simulink model "ofdmexample1"  (R2017a)
settings: Solver=FixedStepDiscrete  StartTime=0.0  StopTime=inf  RelTol=1e-3
PostLoadFcn:
  | prm80216d.blkh = []; prm80216d.action = 'init';
  | commwman80216d_init(prm80216d.blkh, prm80216d.action);
  | if isempty(ans), clear ans; end
StartFcn:
  | if isempty(ans), clear ans; end
libraries: commwman80216d_lib x20, dspsigops x16, commcnvcod2 x7, dspsolvers x2, simulink x2, commrflib2 x2, commdigbbndpm3 x1, commblksprivate x1, commofdm x1, commrandsrc3 x1, commsdrhw_v2 x1
Description:
  | IEEE 802.16-2004 WirelessMAN-OFDM PHY Downlink model
settings Model: FPTRunName=Active  ExtModeAutoUpdateStatusClock=off  Creator=The MathWorks, Inc.  LastModifiedBy=max
settings DataIOCC: LimitDataPoints=on  SaveFormat=Array
settings OptimizationCC: ExpressionDepthLimit=2147483647  InitFltsAndDblsToZero=on  EfficientMapNaN2IntZero=off  LifeSpan=inf
settings DebuggingCC: UnderspecifiedInitializationDetection=Classic  MergeDetectMultiDrivingBlocksExec=none  FcnCallInpInsideContextMsg=warning  AllowSymbolicDim=off  StateNameClashWarn=warning  SFUnexpectedBacktrackingDiag=warning  SFNoUnconditionalDefaultTransitionDiag=warning  SFExecutionAtInitializationDiag=none
settings HardwareCC: ProdBitPerPointer=32  ProdBitPerSizeT=32  ProdBitPerPtrDiffT=32  ProdLargestAtomicFloat=None  ProdIntDivRoundTo=Undefined  ProdEndianess=Unspecified  ProdWordSize=32  ProdHWDeviceType=32-bit Generic
settings ModelReferenceCC: PropagateSignalLabelsOutOfModel=off
settings RTWCC: RetainRTWFile=on
settings GRTTargetCC: TargetFcnLib=ansi_tfl_tmw_new.mat  TargetLangStandard=C89/C90 (ANSI)  GeneratePreprocessorConditionals=Disable all  CombineOutputUpdateFcns=off  GRTInterface=on
settings ConfigComp: CovMetricSettings=dw  CovHtmlReporting=on  CovSaveCumulativeToWorkspaceVar=on  CovSaveSingleToWorkspaceVar=on  CovExternalEMLEnable=off  CovSFcnEnable=off

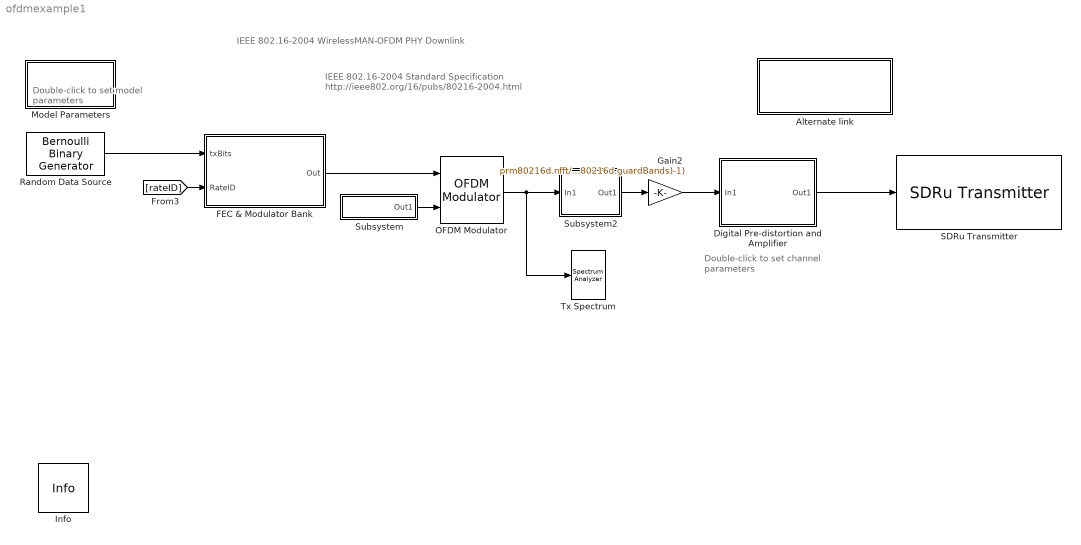
== system ofdmexample1 ==
  note: IEEE 802.16-2004 WirelessMAN-OFDM PHY Downlink
  note: Double-click to set
      | channel parameters
  note: Double-click to
      | set model parameters
  note: IEEE 802.16-2004 Standard Specification
      | http://ieee802.org/16/pubs/80216-2004.html
  Alternate link : Subsystem
      settings: OpenFcn=commwman80216dstbc;
      mask Display: disp('Double-click to open\n link model with\nSpace-Time Block Coding');
  Digital Pre-distortion and Amplifier : Subsystem
      mask Display: disp('Digital\nPre-Distortion and\nNonlinear\nAmplifier')
  FEC & Modulator Bank : Subsystem
      mask Display: disp('FEC & \nModulator Bank');
  Gain2 : Gain  Gain=prm80216d.nfft/sqrt(prm80216d.nfft-sum(prm80216d.guardBands)-1)
  Info : commblksprivate/Info  SystemSampleTime=-1
      settings: SourceProductName=Communications System Toolbox  SourceProductBaseCode=CM
  Model Parameters : Subsystem  mask(Model Parameters){chanBW=3.5, numSym=1, g=1/8, nonlinCtrl=Disabled, dpdCtrl=Disabled, thresh=[4 10 12 19 22 28]}
      mask prompts: chanBW "Channel bandwidth (MHz):"; numSym "Number of OFDM symbols per burst:"; g "Cyclic prefix factor (G):"; nonlinCtrl "Amplifier nonlinearity:"; dpdCtrl "Digital pre-distortion:"; thresh "Low SNR thresholds for rate control (dB):"
      mask help: Specifies model parameters for a simulation run.
      mask init:
      | numPreSym = 1; % number of preamble OFDM symbols
      | 
      | % If the nonlinearity is turned off, then turn off the digital
      | % pre-distortion
      | if nonlinCtrl == 1  % disabled
      |     dpdCtrl = 1;
      | end
      | 
      | myException = commwman80216d_init(gcbh, 'init', chanBW, ...
      |     numSym, numPreSym, g, thresh);
      | 
      | if ~isempty(myException)
      |     errordlg(myException.msg);
      | end
      mask Help: helpview(commdhelp);
      mask TypeOptions g: 1/4 | 1/8 | 1/16 | 1/32
      mask TypeOptions nonlinCtrl: Disabled | Moderate (correctable by pre-distortion) | Severe (uncorrectable by pre-distortion)
      mask Callback nonlinCtrl: commwman80216d_init(gcbh, 'cbShowHidePreDistortion');
      mask TypeOptions dpdCtrl: Disabled | Enabled
      mask Display: disp('Model\nParameters');
  OFDM Modulator : commofdm/OFDM Modulator  FFTLength=prm80216d.nfft  NumGuardBandCarriers=prm80216d.guardBands  InsertDCNull=on  PilotInputPort=on  PilotCarrierIndices=prm80216d.pilotIndices + prm80216d.nfft/2 + 1  CyclicPrefixLength=prm80216d.CPLen  Windowing=off  WindowLength=1  NumSymbols=prm80216d.numOFDMSymbols  NumTransmitAntennas=1  SimulateUsing=Interpreted execution
      settings: SourceProductName=Communications System Toolbox  SourceProductBaseCode=CM
  Random Data Source : commrandsrc3/Bernoulli Binary Generator  ProbabilityOfZero=0.5  SeedSource=Parameter  Seed=61  SampleTime=prm80216d.minBitPeriod  SamplesPerFrame=prm80216d.maxUncBitsPerBlk*prm80216d.numOFDMSymbols  OutputDataType=boolean  SimulateUsing=Interpreted execution
  SDRu Transmitter : commsdrhw_v2/SDRu Transmitter  SourceLibraryInfo="This block requires <a href=\"http://www.mathworks.com/hardware-support/usrp.html\">Communications System Toolbox Support Package for USRP Radio</a>"  rxtx=tx  platform=B210  USRP2_IP='192.168.10.2'  USRP_IP_X300='192.168.10.2'  USRP_IP_X310='192.168.10.2'  USRP_serialNumB200=''  USRP_serialNumB210='30D0D1D'  ChannelMapping=1  centerFrequency=2.484e9  centerFrequencySrc=Dialog  loOffset=0  loOffsetSrc=Dialog  PPSSource=Internal  clockSource=Internal  masterClkRateB200=32e6  masterClkRateB210=8e6  masterClkRateX300=200e6  masterClkRateX310=200e6  masterClkRateParam=8000000  gain=70  gainSrc=Dialog  decimInterp=512  decimInterpSrc=Dialog  TransportDataType=int16  USRP2_IP_NUM=[51 48 68 48 68 49 68]  frameLength=362  outputDatatype=Same as transport data type  overrunUnderrunPort=off  sampleTime=1  dboardInfo=|  HOST_DATA_PORT=30000  HOST_CONTROL_PORT=30001  USRP2_DATA_PORT=32769  USRP2_CONTROL_PORT=32768  bufferMode=Continuous streaming  EnableBurstMode=off  NumFramesInBurst=100  USRP_ID='30D0D1D'
      | dbid: 0
      |           dbName: 'no db found'
      |          freqMin: 0
      |          freqMax: 0
      |          gainMin: 0
      |          gainMax: 0
      |     gainStepSize: 0
      settings: SourceProductName=Communications System Toolbox Support Package for USRP(R) Radio  SourceProductBaseCode=USRP
  Subsystem : Subsystem
      mask Display: disp('Pilot')
  Subsystem2 : Subsystem
      mask Display: disp('Preamble\nPacking');
  Tx Spectrum : SpectrumAnalyzer
  wires:
  Gain2/1 -> Digital Pre-distortion and Amplifier/1(In1)
  Random Data Source/1 -> FEC & Modulator Bank/1(txBits)
  [rateID] -> FEC & Modulator Bank/2(RateID)
  Subsystem/1(Out1) -> OFDM Modulator/2
  OFDM Modulator/1 -> Subsystem2/1(In1), Tx Spectrum/1
  FEC & Modulator Bank/1(Out) -> OFDM Modulator/1
  Subsystem2/1(Out1) -> Gain2/1
  Digital Pre-distortion and Amplifier/1(Out1) -> SDRu Transmitter/1

== system ofdmexample1/Alternate link ==

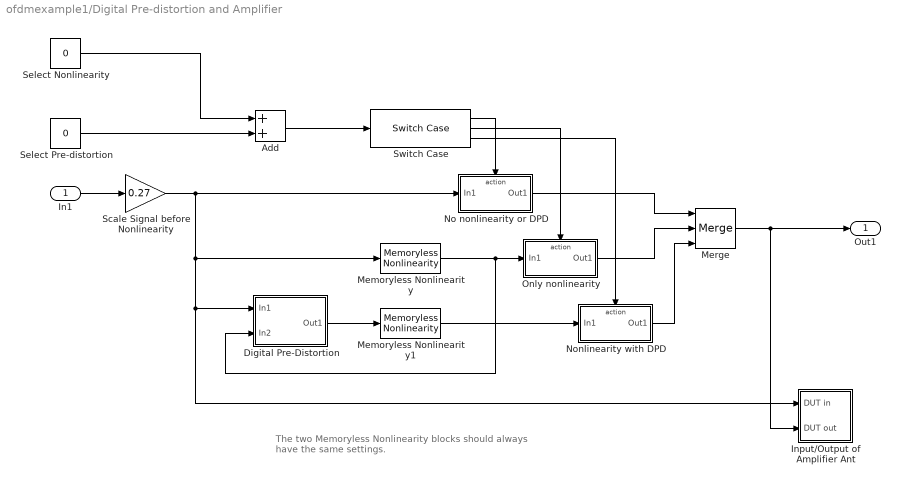
== system ofdmexample1/Digital Pre-distortion and Amplifier ==
  note: The two Memoryless Nonlinearity blocks should always
      | have the same settings.
  In1 : Inport
  Add : Sum
  Digital Pre-Distortion : Subsystem
      mask Display: disp('Digital\nPre-Distortion')
  Input/Output of Amplifier Ant : Subsystem
  Memoryless Nonlinearity : commrflib2/Memoryless Nonlinearity  model_select=Saleh model  linGaindB=0  GindB=0  iip3=30  am2pm=10  LPwrLimAMPM=10  UPwrLimAMPM=inf  amam=[2.1587 1.1517]  ampm=[4.0033 9.1040]  x=[8.1081 1.5413 6.5202 -0.0718]  y=[4.6645 2.0965 10.88 -0.003]  p=0.5  GoutdB=0  vsat=1
      settings: SourceProductName=Communications System Toolbox  SourceProductBaseCode=CM
  Memoryless Nonlinearity1 : commrflib2/Memoryless Nonlinearity  model_select=Saleh model  linGaindB=0  GindB=0  iip3=30  am2pm=10  LPwrLimAMPM=10  UPwrLimAMPM=inf  amam=[2.1587 1.1517]  ampm=[4.0033 9.1040]  x=[8.1081 1.5413 6.5202 -0.0718]  y=[4.6645 2.0965 10.88 -0.003]  p=0.5  GoutdB=0  vsat=1
      settings: SourceProductName=Communications System Toolbox  SourceProductBaseCode=CM
  Merge : Merge  Inputs=3
  No nonlinearity or DPD : Subsystem  TreatAsAtomicUnit=on
  Nonlinearity with DPD : Subsystem  TreatAsAtomicUnit=on
  Only nonlinearity : Subsystem  TreatAsAtomicUnit=on
  Scale Signal before Nonlinearity : Gain  Gain=0.27
  Select Nonlinearity : Constant  Value=0
  Select Pre-distortion : Constant  Value=0
  Switch Case : SwitchCase  CaseConditions={0,1,2}  ShowDefaultCase=off
  Out1 : Outport
  wires:
  Scale Signal before Nonlinearity/1 -> No nonlinearity or DPD/1(In1), Input/Output of Amplifier Ant/1(DUT in), Digital Pre-Distortion/1(In1), Memoryless Nonlinearity/1
  Digital Pre-Distortion/1(Out1) -> Memoryless Nonlinearity1/1
  Select Pre-distortion/1 -> Add/2
  Add/1 -> Switch Case/1
  Select Nonlinearity/1 -> Add/1
  In1/1 -> Scale Signal before Nonlinearity/1
  Memoryless Nonlinearity1/1 -> Nonlinearity with DPD/1(In1)
  Memoryless Nonlinearity/1 -> Only nonlinearity/1(In1), Digital Pre-Distortion/2(In2)
  Merge/1 -> Input/Output of Amplifier Ant/2(DUT out), Out1/1
  Switch Case/1 -> No nonlinearity or DPD/Action
  Switch Case/2 -> Only nonlinearity/Action
  Switch Case/3 -> Nonlinearity with DPD/Action
  No nonlinearity or DPD/1(Out1) -> Merge/1
  Only nonlinearity/1(Out1) -> Merge/2
  Nonlinearity with DPD/1(Out1) -> Merge/3

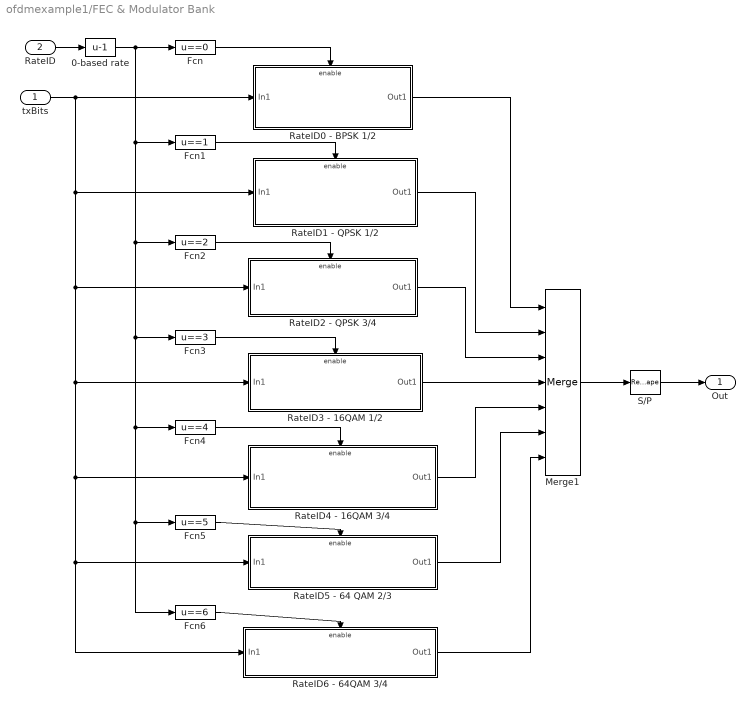
== system ofdmexample1/FEC & Modulator Bank ==
  txBits : Inport
  RateID : Inport  Port=2
  0-based rate : Bias  Bias=-1
  Fcn : Fcn  Expr=u==0
  Fcn1 : Fcn  Expr=u==1
  Fcn2 : Fcn  Expr=u==2
  Fcn3 : Fcn  Expr=u==3
  Fcn4 : Fcn  Expr=u==4
  Fcn5 : Fcn  Expr=u==5
  Fcn6 : Fcn  Expr=u==6
  Merge1 : Merge  Inputs=7
  RateID0 - BPSK 1/2 : Subsystem
  RateID1 - QPSK 1/2 : Subsystem
  RateID2 - QPSK 3/4 : Subsystem
  RateID3 - 16QAM 1/2 : Subsystem
  RateID4 - 16QAM 3/4 : Subsystem
  RateID5 - 64 QAM 2/3 : Subsystem
  RateID6 - 64QAM 3/4 : Subsystem
  S/P : Reshape  OutputDimensionality=Customize  OutputDimensions=[prm80216d.numDataCarriers, prm80216d.numOFDMSymbols]
  Out : Outport
  wires:
  RateID0 - BPSK 1/2/1(Out1) -> Merge1/1
  RateID1 - QPSK 1/2/1(Out1) -> Merge1/2
  RateID2 - QPSK 3/4/1(Out1) -> Merge1/3
  RateID3 - 16QAM 1/2/1(Out1) -> Merge1/4
  RateID4 - 16QAM 3/4/1(Out1) -> Merge1/5
  RateID5 - 64 QAM 2/3/1(Out1) -> Merge1/6
  RateID6 - 64QAM 3/4/1(Out1) -> Merge1/7
  txBits/1 -> RateID5 - 64 QAM 2/3/1(In1), RateID6 - 64QAM 3/4/1(In1), RateID4 - 16QAM 3/4/1(In1), RateID3 - 16QAM 1/2/1(In1), RateID2 - QPSK 3/4/1(In1), RateID1 - QPSK 1/2/1(In1), RateID0 - BPSK 1/2/1(In1)
  RateID/1 -> 0-based rate/1
  Fcn/1 -> RateID0 - BPSK 1/2/Enable
  Fcn1/1 -> RateID1 - QPSK 1/2/Enable
  Fcn2/1 -> RateID2 - QPSK 3/4/Enable
  Fcn3/1 -> RateID3 - 16QAM 1/2/Enable
  Fcn4/1 -> RateID4 - 16QAM 3/4/Enable
  Fcn5/1 -> RateID5 - 64 QAM 2/3/Enable
  Fcn6/1 -> RateID6 - 64QAM 3/4/Enable
  0-based rate/1 -> Fcn4/1, Fcn5/1, Fcn6/1, Fcn3/1, Fcn2/1, Fcn1/1, Fcn/1
  Merge1/1 -> S/P/1
  S/P/1 -> Out/1

== system ofdmexample1/Model Parameters ==
  note: This subsystem is empty.
      | It is used for setting parameter values (in the mask).

== system ofdmexample1/Subsystem ==
  Gain{,1,3..4} (4 alike) : Gain  Gain=-1
  Input Packing : Concatenate  NumInputs=8  Mode=Multidimensional array
  Pilots : commwman80216d_lib/Pilot Generator  link=Downlink  ts=prm80216d.maxUncBitsPerBlk*prm80216d.minBitPeriod  numSym=prm80216d.numOFDMSymbols  shift=prm80216d.numPreamOFDMSymbols
      settings: SourceProductName=Communications System Toolbox  SourceProductBaseCode=CM
  Out1 : Outport
  wires:
  Gain/1 -> Input Packing/4
  Pilots/1 -> Input Packing/1, Gain1/1, Input Packing/3, Gain/1, Gain3/1, Gain4/1, Input Packing/7, Input Packing/8
  Gain3/1 -> Input Packing/5
  Gain1/1 -> Input Packing/2
  Gain4/1 -> Input Packing/6
  Input Packing/1 -> Out1/1

== system ofdmexample1/Subsystem2 ==
  In1 : Inport
  Insert Preamble : Concatenate  Mode=Multidimensional array
  Subsystem1 : Subsystem
      mask Display: disp('Preamble')
  Out1 : Outport
  wires:
  In1/1 -> Insert Preamble/2
  Insert Preamble/1 -> Out1/1
  Subsystem1/1(Out) -> Insert Preamble/1

== system ofdmexample1/Digital Pre-distortion and Amplifier/Digital Pre-Distortion ==
  In1 : Inport
  In2 : Inport  Port=2
  Distortion compensation : Subsystem
  Parameter Estimation : Subsystem
  Out1 : Outport
  wires:
  In1/1 -> Distortion compensation/3(In), Parameter Estimation/1(DUT Input)
  Parameter Estimation/1(c) -> Distortion compensation/1(c)
  Parameter Estimation/2(d) -> Distortion compensation/2(d)
  Distortion compensation/1(Pre-distorted Signal) -> Out1/1
  In2/1 -> Parameter Estimation/2(DUT Output)

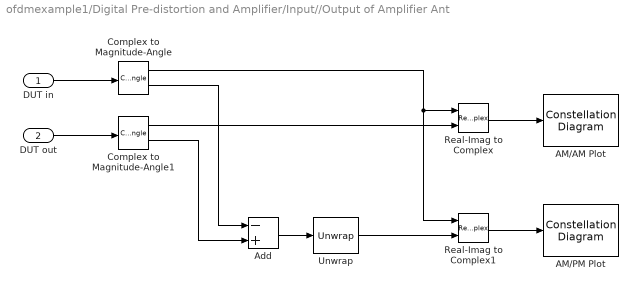
== system ofdmexample1/Digital Pre-distortion and Amplifier/Input//Output of Amplifier Ant ==
  DUT in : Inport
  DUT out : Inport  Port=2
  AM/AM Plot : ConstellationDiagram  Tag=ScatterPlot
  AM/PM Plot : ConstellationDiagram  Tag=ScatterPlot
  Add : Sum  Inputs=-+
  Complex to Magnitude-Angle : ComplexToMagnitudeAngle
  Complex to Magnitude-Angle1 : ComplexToMagnitudeAngle
  Real-Imag to Complex : RealImagToComplex
  Real-Imag to Complex1 : RealImagToComplex
  Unwrap : dspsigops/Unwrap  tol=pi  InputProcessing=Columns as channels (frame based)  running=on
  wires:
  Complex to Magnitude-Angle/1 -> Real-Imag to Complex/1, Real-Imag to Complex1/1
  Complex to Magnitude-Angle1/1 -> Real-Imag to Complex/2
  Real-Imag to Complex/1 -> AM/AM Plot/1
  Real-Imag to Complex1/1 -> AM/PM Plot/1
  DUT in/1 -> Complex to Magnitude-Angle/1
  DUT out/1 -> Complex to Magnitude-Angle1/1
  Complex to Magnitude-Angle1/2 -> Add/2
  Complex to Magnitude-Angle/2 -> Add/1
  Add/1 -> Unwrap/1
  Unwrap/1 -> Real-Imag to Complex1/2

== system ofdmexample1/Digital Pre-distortion and Amplifier/No nonlinearity or DPD ==
  In1 : Inport
  Action Port : ActionPort  ActionType=case
  Out1 : Outport
  wires:
  In1/1 -> Out1/1

== system ofdmexample1/Digital Pre-distortion and Amplifier/Nonlinearity with DPD ==
  In1 : Inport
  Action Port : ActionPort  ActionType=case
  Out1 : Outport
  wires:
  In1/1 -> Out1/1

== system ofdmexample1/Digital Pre-distortion and Amplifier/Only nonlinearity ==
  In1 : Inport
  Action Port : ActionPort  ActionType=case
  Out1 : Outport
  wires:
  In1/1 -> Out1/1

== system ofdmexample1/FEC & Modulator Bank/RateID0 - BPSK 1//2 ==
  In1 : Inport
  Enable : EnablePort  PropagateVarSize=During execution
  BPSK Modulator : commdigbbndpm3/BPSK Modulator Baseband  Ph=0  outDtype=double  outWordLen=16  outUDDataType=sfix(16)  outFracLenMode=Best precision  outFracLen=15  outDataTypeStr=double  outLastDataTypeStr=double
  Convolutional Encoder : commcnvcod2/Convolutional Encoder  trellis=poly2trellis(7, [171 133])  opMode=Truncated (reset every frame)  DelayedResetAction=off  hasIniStPort=off  hasFinStPort=off  usePuncVector=off  punctureVector=[1 0 1]  reset=Unused parameter value
      settings: SourceProductName=Communications System Toolbox  SourceProductBaseCode=CM
  Interleaver : commwman80216d_lib/Interleaver  numSubCh=16  Ncbps1=192  Ncbps2=96  Ncbps3=48  Ncbps4=96  Ncbps5=12  Ncpc=1  numSym=prm80216d.numOFDMSymbols
      settings: SourceProductName=Communications System Toolbox  SourceProductBaseCode=CM
  Select Bits : dspsigops/Pad  padAlong=Columns  dimsToPad=1  valSrc=Specify via dialog  padVal=0  spec=Output size  padNumOutRowsSpecMethod=User-specified  numOutRows=prm80216d.uncBlkSize(1)*8*prm80216d.numOFDMSymbols - 8  padNumOutColsSpecMethod=User-specified  numOutCols=1  isVarDimsMode=off  padBeginning=0  padEnd=0  outSizeMode=User-specified  outSize=1  padSigAt=End  trunc_flag=None  roundingMode=Floor  overflowMode=off  truncOrWrapMode=Truncate  wrap_flag=None
      settings: AttributesFormatString=\n  SourceProductName=DSP System Toolbox  SourceProductBaseCode=DS
  Zero pad tail byte : dspsigops/Pad  padAlong=Columns  dimsToPad=1  valSrc=Specify via dialog  padVal=0  spec=Output size  padNumOutRowsSpecMethod=User-specified  numOutRows=prm80216d.uncBlkSize(1)*8*prm80216d.numOFDMSymbols  padNumOutColsSpecMethod=User-specified  numOutCols=1  isVarDimsMode=off  padBeginning=0  padEnd=0  outSizeMode=User-specified  outSize=1  padSigAt=End  trunc_flag=None  roundingMode=Floor  overflowMode=off  truncOrWrapMode=Truncate  wrap_flag=None
      settings: AttributesFormatString=\n  SourceProductName=DSP System Toolbox  SourceProductBaseCode=DS
  Out1 : Outport
  wires:
  Convolutional Encoder/1 -> Interleaver/1
  Interleaver/1 -> BPSK Modulator/1
  In1/1 -> Select Bits/1
  BPSK Modulator/1 -> Out1/1
  Select Bits/1 -> Zero pad tail byte/1
  Zero pad tail byte/1 -> Convolutional Encoder/1

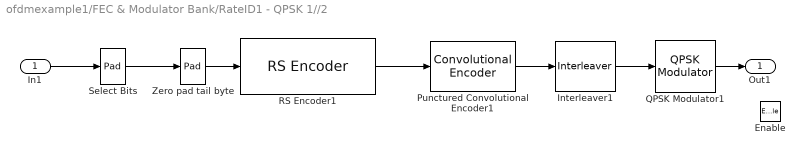
== system ofdmexample1/FEC & Modulator Bank/RateID1 - QPSK 1//2 ==
  In1 : Inport
  Enable : EnablePort  PropagateVarSize=During execution
  Interleaver1 : commwman80216d_lib/Interleaver  numSubCh=16  Ncbps1=384  Ncbps2=96  Ncbps3=48  Ncbps4=96  Ncbps5=12  Ncpc=2  numSym=prm80216d.numOFDMSymbols
      settings: SourceProductName=Communications System Toolbox  SourceProductBaseCode=CM
  Punctured Convolutional Encoder1 : commcnvcod2/Convolutional Encoder  trellis=poly2trellis(7, [171 133])  opMode=Truncated (reset every frame)  DelayedResetAction=off  hasIniStPort=off  hasFinStPort=off  usePuncVector=on  punctureVector=reshape([1 0;1 1],4,1)  reset=Unused parameter value
      settings: SourceProductName=Communications System Toolbox  SourceProductBaseCode=CM
  QPSK Modulator1 : commwman80216d_lib/QPSK Modulator  SystemSampleTime=-1
      settings: SourceProductName=Communications System Toolbox  SourceProductBaseCode=CM
  RS Encoder1 : commwman80216d_lib/RS Encoder  N=32  K=24  numSym=prm80216d.numOFDMSymbols
      settings: SourceProductName=Communications System Toolbox  SourceProductBaseCode=CM
  Select Bits : dspsigops/Pad  padAlong=Columns  dimsToPad=1  valSrc=Specify via dialog  padVal=0  spec=Output size  padNumOutRowsSpecMethod=User-specified  numOutRows=prm80216d.uncBlkSize(2)*8*prm80216d.numOFDMSymbols - 8  padNumOutColsSpecMethod=User-specified  numOutCols=1  isVarDimsMode=off  padBeginning=0  padEnd=0  outSizeMode=User-specified  outSize=1  padSigAt=End  trunc_flag=None  roundingMode=Floor  overflowMode=off  truncOrWrapMode=Truncate  wrap_flag=None
      settings: AttributesFormatString=\n  SourceProductName=DSP System Toolbox  SourceProductBaseCode=DS
  Zero pad tail byte : dspsigops/Pad  padAlong=Columns  dimsToPad=1  valSrc=Specify via dialog  padVal=0  spec=Output size  padNumOutRowsSpecMethod=User-specified  numOutRows=prm80216d.uncBlkSize(2)*8*prm80216d.numOFDMSymbols  padNumOutColsSpecMethod=User-specified  numOutCols=1  isVarDimsMode=off  padBeginning=0  padEnd=0  outSizeMode=User-specified  outSize=1  padSigAt=End  trunc_flag=None  roundingMode=Floor  overflowMode=off  truncOrWrapMode=Truncate  wrap_flag=None
      settings: AttributesFormatString=\n  SourceProductName=DSP System Toolbox  SourceProductBaseCode=DS
  Out1 : Outport
  wires:
  RS Encoder1/1 -> Punctured Convolutional Encoder1/1
  Punctured Convolutional Encoder1/1 -> Interleaver1/1
  Interleaver1/1 -> QPSK Modulator1/1
  In1/1 -> Select Bits/1
  QPSK Modulator1/1 -> Out1/1
  Select Bits/1 -> Zero pad tail byte/1
  Zero pad tail byte/1 -> RS Encoder1/1

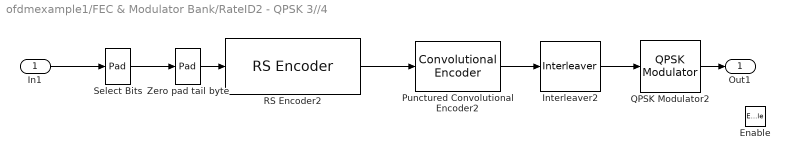
== system ofdmexample1/FEC & Modulator Bank/RateID2 - QPSK 3//4 ==
  In1 : Inport
  Enable : EnablePort  PropagateVarSize=During execution
  Interleaver2 : commwman80216d_lib/Interleaver  numSubCh=16  Ncbps1=384  Ncbps2=96  Ncbps3=48  Ncbps4=96  Ncbps5=12  Ncpc=2  numSym=prm80216d.numOFDMSymbols
      settings: SourceProductName=Communications System Toolbox  SourceProductBaseCode=CM
  Punctured Convolutional Encoder2 : commcnvcod2/Convolutional Encoder  trellis=poly2trellis(7, [171 133])  opMode=Truncated (reset every frame)  DelayedResetAction=off  hasIniStPort=off  hasFinStPort=off  usePuncVector=on  punctureVector=reshape([1 0 1 0 1;1 1 0 1 0],10,1)  reset=Unused parameter value
      settings: SourceProductName=Communications System Toolbox  SourceProductBaseCode=CM
  QPSK Modulator2 : commwman80216d_lib/QPSK Modulator  SystemSampleTime=-1
      settings: SourceProductName=Communications System Toolbox  SourceProductBaseCode=CM
  RS Encoder2 : commwman80216d_lib/RS Encoder  N=40  K=36  numSym=prm80216d.numOFDMSymbols
      settings: SourceProductName=Communications System Toolbox  SourceProductBaseCode=CM
  Select Bits : dspsigops/Pad  padAlong=Columns  dimsToPad=1  valSrc=Specify via dialog  padVal=0  spec=Output size  padNumOutRowsSpecMethod=User-specified  numOutRows=prm80216d.uncBlkSize(3)*8*prm80216d.numOFDMSymbols - 8  padNumOutColsSpecMethod=User-specified  numOutCols=1  isVarDimsMode=off  padBeginning=0  padEnd=0  outSizeMode=User-specified  outSize=1  padSigAt=End  trunc_flag=None  roundingMode=Floor  overflowMode=off  truncOrWrapMode=Truncate  wrap_flag=None
      settings: AttributesFormatString=\n  SourceProductName=DSP System Toolbox  SourceProductBaseCode=DS
  Zero pad tail byte : dspsigops/Pad  padAlong=Columns  dimsToPad=1  valSrc=Specify via dialog  padVal=0  spec=Output size  padNumOutRowsSpecMethod=User-specified  numOutRows=prm80216d.uncBlkSize(3)*8*prm80216d.numOFDMSymbols  padNumOutColsSpecMethod=User-specified  numOutCols=1  isVarDimsMode=off  padBeginning=0  padEnd=0  outSizeMode=User-specified  outSize=1  padSigAt=End  trunc_flag=None  roundingMode=Floor  overflowMode=off  truncOrWrapMode=Truncate  wrap_flag=None
      settings: AttributesFormatString=\n  SourceProductName=DSP System Toolbox  SourceProductBaseCode=DS
  Out1 : Outport
  wires:
  RS Encoder2/1 -> Punctured Convolutional Encoder2/1
  Punctured Convolutional Encoder2/1 -> Interleaver2/1
  Interleaver2/1 -> QPSK Modulator2/1
  In1/1 -> Select Bits/1
  QPSK Modulator2/1 -> Out1/1
  Select Bits/1 -> Zero pad tail byte/1
  Zero pad tail byte/1 -> RS Encoder2/1

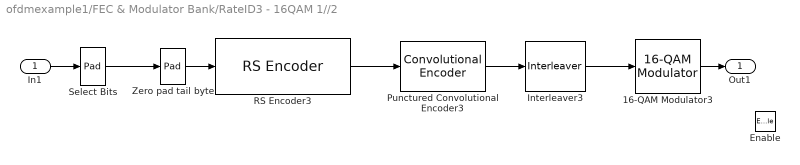
== system ofdmexample1/FEC & Modulator Bank/RateID3 - 16QAM 1//2 ==
  In1 : Inport
  Enable : EnablePort  PropagateVarSize=During execution
  16-QAM Modulator3 : commwman80216d_lib/16-QAM Modulator  SystemSampleTime=-1
      settings: SourceProductName=Communications System Toolbox  SourceProductBaseCode=CM
  Interleaver3 : commwman80216d_lib/Interleaver  numSubCh=16  Ncbps1=768  Ncbps2=96  Ncbps3=48  Ncbps4=96  Ncbps5=12  Ncpc=4  numSym=prm80216d.numOFDMSymbols
      settings: SourceProductName=Communications System Toolbox  SourceProductBaseCode=CM
  Punctured Convolutional Encoder3 : commcnvcod2/Convolutional Encoder  trellis=poly2trellis(7, [171 133])  opMode=Truncated (reset every frame)  DelayedResetAction=off  hasIniStPort=off  hasFinStPort=off  usePuncVector=on  punctureVector=reshape([1 0;1 1],4,1)  reset=Unused parameter value
      settings: SourceProductName=Communications System Toolbox  SourceProductBaseCode=CM
  RS Encoder3 : commwman80216d_lib/RS Encoder  N=64  K=48  numSym=prm80216d.numOFDMSymbols
      settings: SourceProductName=Communications System Toolbox  SourceProductBaseCode=CM
  Select Bits : dspsigops/Pad  padAlong=Columns  dimsToPad=1  valSrc=Specify via dialog  padVal=0  spec=Output size  padNumOutRowsSpecMethod=User-specified  numOutRows=prm80216d.uncBlkSize(4)*8*prm80216d.numOFDMSymbols - 8  padNumOutColsSpecMethod=User-specified  numOutCols=1  isVarDimsMode=off  padBeginning=0  padEnd=0  outSizeMode=User-specified  outSize=1  padSigAt=End  trunc_flag=None  roundingMode=Floor  overflowMode=off  truncOrWrapMode=Truncate  wrap_flag=None
      settings: AttributesFormatString=\n  SourceProductName=DSP System Toolbox  SourceProductBaseCode=DS
  Zero pad tail byte : dspsigops/Pad  padAlong=Columns  dimsToPad=1  valSrc=Specify via dialog  padVal=0  spec=Output size  padNumOutRowsSpecMethod=User-specified  numOutRows=prm80216d.uncBlkSize(4)*8*prm80216d.numOFDMSymbols  padNumOutColsSpecMethod=User-specified  numOutCols=1  isVarDimsMode=off  padBeginning=0  padEnd=0  outSizeMode=User-specified  outSize=1  padSigAt=End  trunc_flag=None  roundingMode=Floor  overflowMode=off  truncOrWrapMode=Truncate  wrap_flag=None
      settings: AttributesFormatString=\n  SourceProductName=DSP System Toolbox  SourceProductBaseCode=DS
  Out1 : Outport
  wires:
  RS Encoder3/1 -> Punctured Convolutional Encoder3/1
  Punctured Convolutional Encoder3/1 -> Interleaver3/1
  Interleaver3/1 -> 16-QAM Modulator3/1
  In1/1 -> Select Bits/1
  16-QAM Modulator3/1 -> Out1/1
  Select Bits/1 -> Zero pad tail byte/1
  Zero pad tail byte/1 -> RS Encoder3/1

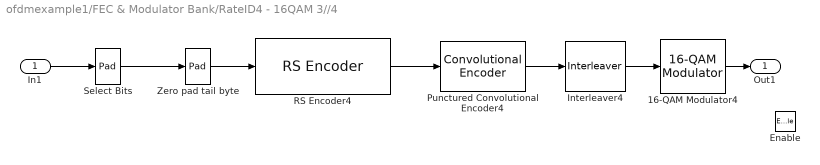
== system ofdmexample1/FEC & Modulator Bank/RateID4 - 16QAM 3//4 ==
  In1 : Inport
  Enable : EnablePort  PropagateVarSize=During execution
  16-QAM Modulator4 : commwman80216d_lib/16-QAM Modulator  SystemSampleTime=-1
      settings: SourceProductName=Communications System Toolbox  SourceProductBaseCode=CM
  Interleaver4 : commwman80216d_lib/Interleaver  numSubCh=16  Ncbps1=768  Ncbps2=96  Ncbps3=48  Ncbps4=96  Ncbps5=12  Ncpc=4  numSym=prm80216d.numOFDMSymbols
      settings: SourceProductName=Communications System Toolbox  SourceProductBaseCode=CM
  Punctured Convolutional Encoder4 : commcnvcod2/Convolutional Encoder  trellis=poly2trellis(7, [171 133])  opMode=Truncated (reset every frame)  DelayedResetAction=off  hasIniStPort=off  hasFinStPort=off  usePuncVector=on  punctureVector=reshape([1 0 1 0 1;1 1 0 1 0],10,1)  reset=Unused parameter value
      settings: SourceProductName=Communications System Toolbox  SourceProductBaseCode=CM
  RS Encoder4 : commwman80216d_lib/RS Encoder  N=80  K=72  numSym=prm80216d.numOFDMSymbols
      settings: SourceProductName=Communications System Toolbox  SourceProductBaseCode=CM
  Select Bits : dspsigops/Pad  padAlong=Columns  dimsToPad=1  valSrc=Specify via dialog  padVal=0  spec=Output size  padNumOutRowsSpecMethod=User-specified  numOutRows=prm80216d.uncBlkSize(5)*8*prm80216d.numOFDMSymbols - 8  padNumOutColsSpecMethod=User-specified  numOutCols=1  isVarDimsMode=off  padBeginning=0  padEnd=0  outSizeMode=User-specified  outSize=1  padSigAt=End  trunc_flag=None  roundingMode=Floor  overflowMode=off  truncOrWrapMode=Truncate  wrap_flag=None
      settings: AttributesFormatString=\n  SourceProductName=DSP System Toolbox  SourceProductBaseCode=DS
  Zero pad tail byte : dspsigops/Pad  padAlong=Columns  dimsToPad=1  valSrc=Specify via dialog  padVal=0  spec=Output size  padNumOutRowsSpecMethod=User-specified  numOutRows=prm80216d.uncBlkSize(5)*8*prm80216d.numOFDMSymbols  padNumOutColsSpecMethod=User-specified  numOutCols=1  isVarDimsMode=off  padBeginning=0  padEnd=0  outSizeMode=User-specified  outSize=1  padSigAt=End  trunc_flag=None  roundingMode=Floor  overflowMode=off  truncOrWrapMode=Truncate  wrap_flag=None
      settings: AttributesFormatString=\n  SourceProductName=DSP System Toolbox  SourceProductBaseCode=DS
  Out1 : Outport
  wires:
  RS Encoder4/1 -> Punctured Convolutional Encoder4/1
  Punctured Convolutional Encoder4/1 -> Interleaver4/1
  Interleaver4/1 -> 16-QAM Modulator4/1
  In1/1 -> Select Bits/1
  16-QAM Modulator4/1 -> Out1/1
  Select Bits/1 -> Zero pad tail byte/1
  Zero pad tail byte/1 -> RS Encoder4/1

== system ofdmexample1/FEC & Modulator Bank/RateID5 - 64 QAM 2//3 ==
  In1 : Inport
  Enable : EnablePort  PropagateVarSize=During execution
  64-QAM Modulator5 : commwman80216d_lib/64-QAM Modulator  SystemSampleTime=-1
      settings: SourceProductName=Communications System Toolbox  SourceProductBaseCode=CM
  Interleaver5 : commwman80216d_lib/Interleaver  numSubCh=16  Ncbps1=1152  Ncbps2=96  Ncbps3=48  Ncbps4=96  Ncbps5=12  Ncpc=6  numSym=prm80216d.numOFDMSymbols
      settings: SourceProductName=Communications System Toolbox  SourceProductBaseCode=CM
  Punctured Convolutional Encoder5 : commcnvcod2/Convolutional Encoder  trellis=poly2trellis(7, [171 133])  opMode=Truncated (reset every frame)  DelayedResetAction=off  hasIniStPort=off  hasFinStPort=off  usePuncVector=on  punctureVector=reshape([1 0 1;1 1 0 ],6,1)  reset=Unused parameter value
      settings: SourceProductName=Communications System Toolbox  SourceProductBaseCode=CM
  RS Encoder5 : commwman80216d_lib/RS Encoder  N=108  K=96  numSym=prm80216d.numOFDMSymbols
      settings: SourceProductName=Communications System Toolbox  SourceProductBaseCode=CM
  Select Bits : dspsigops/Pad  padAlong=Columns  dimsToPad=1  valSrc=Specify via dialog  padVal=0  spec=Output size  padNumOutRowsSpecMethod=User-specified  numOutRows=prm80216d.uncBlkSize(6)*8*prm80216d.numOFDMSymbols - 8  padNumOutColsSpecMethod=User-specified  numOutCols=1  isVarDimsMode=off  padBeginning=0  padEnd=0  outSizeMode=User-specified  outSize=1  padSigAt=End  trunc_flag=None  roundingMode=Floor  overflowMode=off  truncOrWrapMode=Truncate  wrap_flag=None
      settings: AttributesFormatString=\n  SourceProductName=DSP System Toolbox  SourceProductBaseCode=DS
  Zero pad tail byte : dspsigops/Pad  padAlong=Columns  dimsToPad=1  valSrc=Specify via dialog  padVal=0  spec=Output size  padNumOutRowsSpecMethod=User-specified  numOutRows=prm80216d.uncBlkSize(6)*8*prm80216d.numOFDMSymbols  padNumOutColsSpecMethod=User-specified  numOutCols=1  isVarDimsMode=off  padBeginning=0  padEnd=0  outSizeMode=User-specified  outSize=1  padSigAt=End  trunc_flag=None  roundingMode=Floor  overflowMode=off  truncOrWrapMode=Truncate  wrap_flag=None
      settings: AttributesFormatString=\n  SourceProductName=DSP System Toolbox  SourceProductBaseCode=DS
  Out1 : Outport
  wires:
  RS Encoder5/1 -> Punctured Convolutional Encoder5/1
  Punctured Convolutional Encoder5/1 -> Interleaver5/1
  Interleaver5/1 -> 64-QAM Modulator5/1
  In1/1 -> Select Bits/1
  64-QAM Modulator5/1 -> Out1/1
  Select Bits/1 -> Zero pad tail byte/1
  Zero pad tail byte/1 -> RS Encoder5/1

== system ofdmexample1/FEC & Modulator Bank/RateID6 - 64QAM 3//4 ==
  In1 : Inport
  Enable : EnablePort  PropagateVarSize=During execution
  64-QAM Modulator6 : commwman80216d_lib/64-QAM Modulator  SystemSampleTime=-1
      settings: SourceProductName=Communications System Toolbox  SourceProductBaseCode=CM
  Interleaver6 : commwman80216d_lib/Interleaver  numSubCh=16  Ncbps1=1152  Ncbps2=96  Ncbps3=48  Ncbps4=96  Ncbps5=12  Ncpc=6  numSym=prm80216d.numOFDMSymbols
      settings: SourceProductName=Communications System Toolbox  SourceProductBaseCode=CM
  Punctured Convolutional Encoder6 : commcnvcod2/Convolutional Encoder  trellis=poly2trellis(7, [171 133])  opMode=Truncated (reset every frame)  DelayedResetAction=off  hasIniStPort=off  hasFinStPort=off  usePuncVector=on  punctureVector=reshape([1 0 1 0 1;1 1 0 1 0], 10, 1)  reset=Unused parameter value
      settings: SourceProductName=Communications System Toolbox  SourceProductBaseCode=CM
  RS Encoder6 : commwman80216d_lib/RS Encoder  N=120  K=108  numSym=prm80216d.numOFDMSymbols
      settings: SourceProductName=Communications System Toolbox  SourceProductBaseCode=CM
  Select Bits : dspsigops/Pad  padAlong=Columns  dimsToPad=1  valSrc=Specify via dialog  padVal=0  spec=Output size  padNumOutRowsSpecMethod=User-specified  numOutRows=prm80216d.uncBlkSize(7)*8*prm80216d.numOFDMSymbols - 8  padNumOutColsSpecMethod=User-specified  numOutCols=1  isVarDimsMode=off  padBeginning=0  padEnd=0  outSizeMode=User-specified  outSize=1  padSigAt=End  trunc_flag=None  roundingMode=Floor  overflowMode=off  truncOrWrapMode=Truncate  wrap_flag=None
      settings: AttributesFormatString=\n  SourceProductName=DSP System Toolbox  SourceProductBaseCode=DS
  Zero pad tail byte : dspsigops/Pad  padAlong=Columns  dimsToPad=1  valSrc=Specify via dialog  padVal=0  spec=Output size  padNumOutRowsSpecMethod=User-specified  numOutRows=prm80216d.uncBlkSize(7)*8*prm80216d.numOFDMSymbols  padNumOutColsSpecMethod=User-specified  numOutCols=1  isVarDimsMode=off  padBeginning=0  padEnd=0  outSizeMode=User-specified  outSize=1  padSigAt=End  trunc_flag=None  roundingMode=Floor  overflowMode=off  truncOrWrapMode=Truncate  wrap_flag=None
      settings: AttributesFormatString=\n  SourceProductName=DSP System Toolbox  SourceProductBaseCode=DS
  Out1 : Outport
  wires:
  RS Encoder6/1 -> Punctured Convolutional Encoder6/1
  Punctured Convolutional Encoder6/1 -> Interleaver6/1
  Interleaver6/1 -> 64-QAM Modulator6/1
  In1/1 -> Select Bits/1
  64-QAM Modulator6/1 -> Out1/1
  Select Bits/1 -> Zero pad tail byte/1
  Zero pad tail byte/1 -> RS Encoder6/1

== system ofdmexample1/Subsystem2/Subsystem1 ==
  Modulated Preamble : Constant  Value=prm80216d.modedPreamble  VectorParams1D=off
  Out : Outport
  wires:
  Modulated Preamble/1 -> Out/1

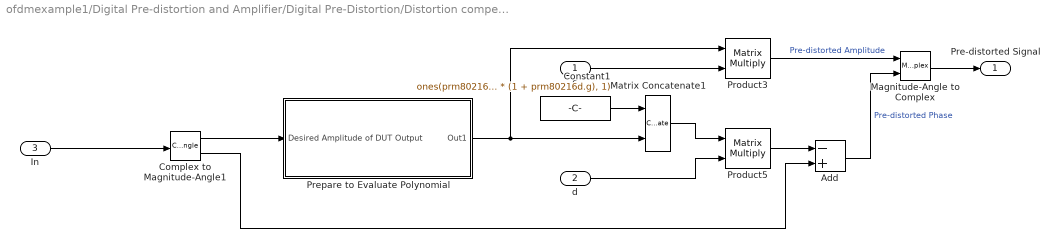
== system ofdmexample1/Digital Pre-distortion and Amplifier/Digital Pre-Distortion/Distortion compensation ==
  c : Inport
  d : Inport  Port=2
  In : Inport  Port=3
  Add : Sum  Inputs=-+
  Complex to Magnitude-Angle1 : ComplexToMagnitudeAngle
  Constant1 : Constant  Value=ones(prm80216d.totOFDMSym * prm80216d.nfft * (1 + prm80216d.g), 1)
  Magnitude-Angle to Complex : MagnitudeAngleToComplex
  Matrix Concatenate1 : Concatenate  Mode=Multidimensional array  ConcatenateDimension=2
  Prepare to Evaluate Polynomial : Subsystem
  Product3 : Product  Multiplication=Matrix(*)  RndMeth=Zero
  Product5 : Product  Multiplication=Matrix(*)  RndMeth=Zero
  Pre-distorted Signal : Outport
  wires:
  c/1 -> Product3/2
  Add/1 -> Magnitude-Angle to Complex/2  "Pre-distorted Phase"
  Product5/1 -> Add/1
  Product3/1 -> Magnitude-Angle to Complex/1  "Pre-distorted Amplitude"
  d/1 -> Product5/2
  In/1 -> Complex to Magnitude-Angle1/1
  Magnitude-Angle to Complex/1 -> Pre-distorted Signal/1
  Complex to Magnitude-Angle1/2 -> Add/2
  Complex to Magnitude-Angle1/1 -> Prepare to Evaluate Polynomial/1(Desired Amplitude of DUT Output)
  Matrix Concatenate1/1 -> Product5/1
  Prepare to Evaluate Polynomial/1(Out1) -> Matrix Concatenate1/2, Product3/1
  Constant1/1 -> Matrix Concatenate1/1

== system ofdmexample1/Digital Pre-distortion and Amplifier/Digital Pre-Distortion/Parameter Estimation ==
  DUT Input : Inport
  DUT Output : Inport  Port=2
  Complex to Magnitude-Angle : ComplexToMagnitudeAngle
  Complex to Magnitude-Angle1 : ComplexToMagnitudeAngle
  Polynomial Approximation : Subsystem
  c : Outport
  d : Outport  Port=2
  wires:
  DUT Input/1 -> Complex to Magnitude-Angle/1
  DUT Output/1 -> Complex to Magnitude-Angle1/1
  Complex to Magnitude-Angle1/1 -> Polynomial Approximation/3(Amplitude of DUT Output)
  Complex to Magnitude-Angle/2 -> Polynomial Approximation/2(Phase of DUT Input)
  Polynomial Approximation/1(Coef_c) -> c/1
  Polynomial Approximation/2(Coef_d) -> d/1
  Complex to Magnitude-Angle1/2 -> Polynomial Approximation/4(Phase of DUT Output)
  Complex to Magnitude-Angle/1 -> Polynomial Approximation/1(Amplitude of DUT Input)

== system ofdmexample1/Digital Pre-distortion and Amplifier/Digital Pre-Distortion/Distortion compensation/Prepare to Evaluate Polynomial ==
  Desired Amplitude of DUT Output : Inport
  Matrix Concatenate1 : Concatenate  NumInputs=5  Mode=Multidimensional array  ConcatenateDimension=2
  Product{6..9} (4 alike) : Product  RndMeth=Zero
  Out1 : Outport
  wires:
  Desired Amplitude of DUT Output/1 -> Product9/2, Product8/2, Product7/2, Product6/2, Product6/1, Matrix Concatenate1/1
  Product7/1 -> Product8/1, Matrix Concatenate1/3
  Product6/1 -> Product7/1, Matrix Concatenate1/2
  Product8/1 -> Product9/1, Matrix Concatenate1/4
  Product9/1 -> Matrix Concatenate1/5
  Matrix Concatenate1/1 -> Out1/1

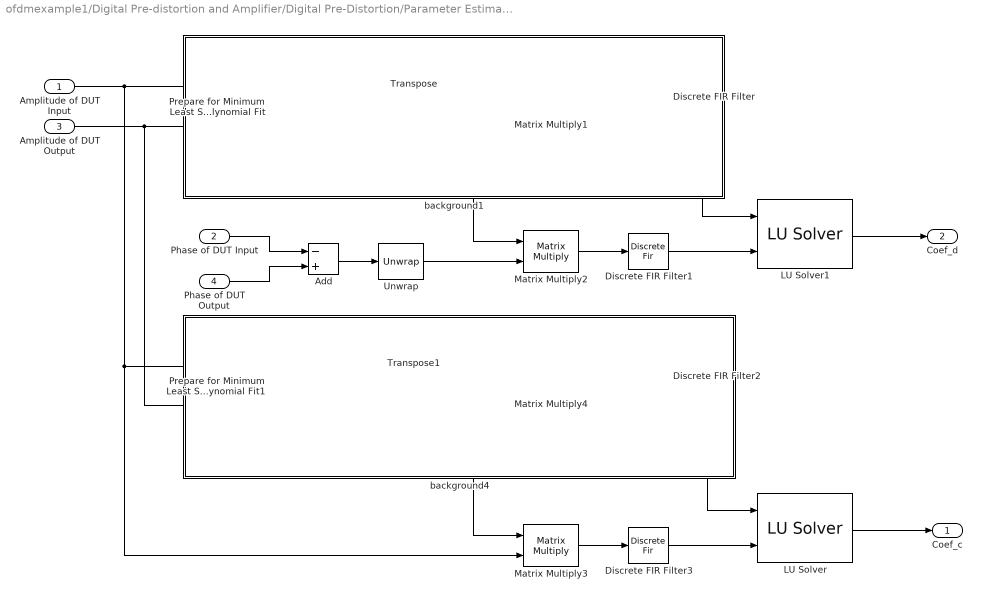
== system ofdmexample1/Digital Pre-distortion and Amplifier/Digital Pre-Distortion/Parameter Estimation/Polynomial Approximation ==
  Amplitude of DUT Input : Inport
  Phase of DUT Input : Inport  Port=2
  Amplitude of DUT Output : Inport  Port=3
  Phase of DUT Output : Inport  Port=4
  Add : Sum  Inputs=-+
  Discrete FIR Filter{,1..3} (4 alike) : DiscreteFir  Coefficients=ones(1,50)  AccumDataTypeStr=Inherit: Same as product output
  LU Solver : dspsolvers/LU Solver
      settings: SourceProductName=DSP System Toolbox  SourceProductBaseCode=DS
  LU Solver1 : dspsolvers/LU Solver
      settings: SourceProductName=DSP System Toolbox  SourceProductBaseCode=DS
  Matrix Multiply{1..4} (4 alike) : Product  Multiplication=Matrix(*)
  Prepare for Minimum Least Square Error Polynomial Fit : Subsystem
  Prepare for Minimum Least Square Error Polynomial Fit1 : Subsystem
  Transpose : Math  Operator=transpose  SaturateOnIntegerOverflow=on
  Transpose1 : Math  Operator=transpose  SaturateOnIntegerOverflow=on
  Unwrap : dspsigops/Unwrap  tol=pi  InputProcessing=Columns as channels (frame based)  running=off
  background1 : Subsystem
      mask Display: disp('')
  background4 : Subsystem
      mask Display: disp('')
  Coef_c : Outport
  Coef_d : Outport  Port=2
  wires:
  Discrete FIR Filter2/1 -> LU Solver/1
  Transpose1/1 -> Matrix Multiply3/1, Matrix Multiply4/1
  Matrix Multiply4/1 -> Discrete FIR Filter2/1
  Prepare for Minimum Least Square Error Polynomial Fit1/1(Out1) -> Matrix Multiply4/2, Transpose1/1
  Phase of DUT Input/1 -> Add/1
  Add/1 -> Unwrap/1
  Amplitude of DUT Input/1 -> Prepare for Minimum Least Square Error Polynomial Fit/1(In1), Prepare for Minimum Least Square Error Polynomial Fit1/1(In1), Matrix Multiply3/2
  Matrix Multiply1/1 -> Discrete FIR Filter/1
  Matrix Multiply3/1 -> Discrete FIR Filter3/1
  Prepare for Minimum Least Square Error Polynomial Fit/1(Out1) -> Matrix Multiply1/2, Transpose/1
  Unwrap/1 -> Matrix Multiply2/2
  Matrix Multiply2/1 -> Discrete FIR Filter1/1
  Amplitude of DUT Output/1 -> Prepare for Minimum Least Square Error Polynomial Fit1/2(In2), Prepare for Minimum Least Square Error Polynomial Fit/2(In2)
  Discrete FIR Filter1/1 -> LU Solver1/2
  Discrete FIR Filter/1 -> LU Solver1/1
  Discrete FIR Filter3/1 -> LU Solver/2
  Phase of DUT Output/1 -> Add/2
  LU Solver1/1 -> Coef_d/1
  LU Solver/1 -> Coef_c/1
  Transpose/1 -> Matrix Multiply1/1, Matrix Multiply2/1

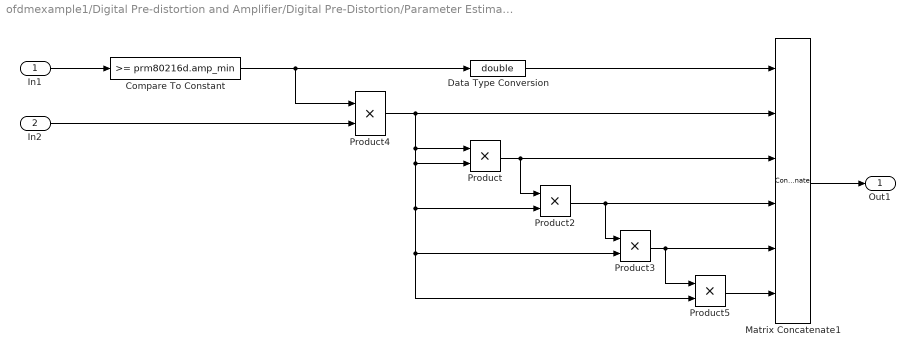
== system ofdmexample1/Digital Pre-distortion and Amplifier/Digital Pre-Distortion/Parameter Estimation/Polynomial Approximation/Prepare for Minimum Least Square Error Polynomial Fit ==
  In1 : Inport
  In2 : Inport  Port=2
  Compare To Constant : simulink/Logic and Bit Operations/Compare To Constant  relop=>=  const=prm80216d.amp_min  OutDataTypeStr=uint8  ZeroCross=off
  Data Type Conversion : DataTypeConversion  OutDataTypeStr=double
  Matrix Concatenate1 : Concatenate  NumInputs=6  Mode=Multidimensional array  ConcatenateDimension=2
  Product{,2..5} (5 alike) : Product  RndMeth=Zero
  Out1 : Outport
  wires:
  Compare To Constant/1 -> Product4/1, Data Type Conversion/1
  In2/1 -> Product4/2
  Product3/1 -> Product5/1, Matrix Concatenate1/5
  Product2/1 -> Product3/1, Matrix Concatenate1/4
  Product/1 -> Product2/1, Matrix Concatenate1/3
  Product4/1 -> Product5/2, Product3/2, Product2/2, Product/2, Product/1, Matrix Concatenate1/2
  Product5/1 -> Matrix Concatenate1/6
  Matrix Concatenate1/1 -> Out1/1
  In1/1 -> Compare To Constant/1
  Data Type Conversion/1 -> Matrix Concatenate1/1

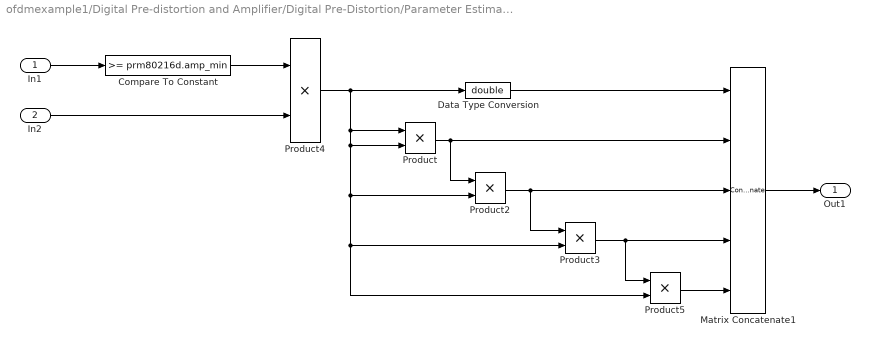
== system ofdmexample1/Digital Pre-distortion and Amplifier/Digital Pre-Distortion/Parameter Estimation/Polynomial Approximation/Prepare for Minimum Least Square Error Polynomial Fit1 ==
  In1 : Inport
  In2 : Inport  Port=2
  Compare To Constant : simulink/Logic and Bit Operations/Compare To Constant  relop=>=  const=prm80216d.amp_min  OutDataTypeStr=uint8  ZeroCross=off
  Data Type Conversion : DataTypeConversion  OutDataTypeStr=double
  Matrix Concatenate1 : Concatenate  NumInputs=5  Mode=Multidimensional array  ConcatenateDimension=2
  Product{,2..5} (5 alike) : Product  RndMeth=Zero
  Out1 : Outport
  wires:
  Compare To Constant/1 -> Product4/1
  Data Type Conversion/1 -> Matrix Concatenate1/1
  In2/1 -> Product4/2
  Product/1 -> Product2/1, Matrix Concatenate1/2
  Product4/1 -> Data Type Conversion/1, Product3/2, Product5/2, Product2/2, Product/2, Product/1
  Product5/1 -> Matrix Concatenate1/5
  Product3/1 -> Matrix Concatenate1/4, Product5/1
  Product2/1 -> Matrix Concatenate1/3, Product3/1
  Matrix Concatenate1/1 -> Out1/1
  In1/1 -> Compare To Constant/1

== system ofdmexample1/Digital Pre-distortion and Amplifier/Digital Pre-Distortion/Parameter Estimation/Polynomial Approximation/background1 ==

== system ofdmexample1/Digital Pre-distortion and Amplifier/Digital Pre-Distortion/Parameter Estimation/Polynomial Approximation/background4 ==
